simulink model "LTI_Unmodeled_test"  (Simulink 7.3)
settings: Solver=ode45  StartTime=0.0  StopTime=10.0  RelTol=1e-3
settings Model: Creator=MD710  LastModifiedBy=MD710
settings DebuggingCC: SaveWithParameterizedLinksMsg=none  SolverPrmCheckMsg=none  MultiTaskDSMMsg=warning  MultiTaskCondExecSysMsg=none  FcnCallInpInsideContextMsg=Enable All  StrictBusMsg=None
settings HardwareCC: TargetHWDeviceType=32-bit Generic
settings RTWCC: IncludeERTFirstTime=on
settings GRTTargetCC: TargetFcnLib=ansi_tfl_tmw.mat

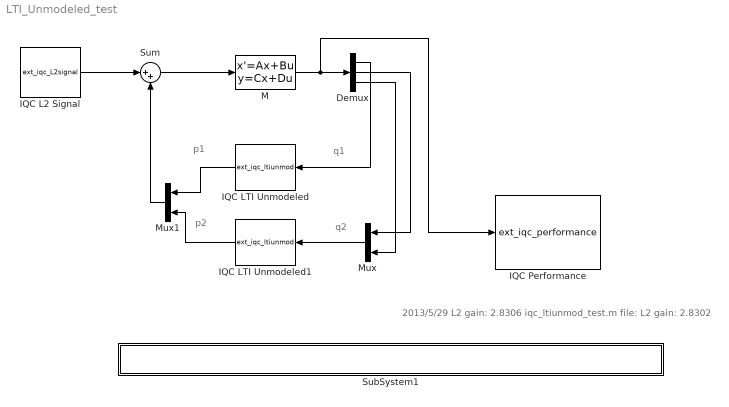
== system LTI_Unmodeled_test ==
  note: p1
  note: q1
  note: q2
  note: p2
  note: 2013/5/29 L2 gain: 2.8306
      | iqc_ltiunmod_test.m file: L2 gain: 2.8302
  Demux : Demux  Outputs=3
  IQC L2 Signal : M-S-Function  FunctionName=ext_iqc_L2signal  Parameters=sig_size,sam_time,sig_type,tru_time,sig_amp,sig_fre,user_cus  mask(IQC L2 signal(ver:0.1)){sig_size=2, sam_time=0, sig_type=Step, tru_time=10, sig_amp=1, sig_fre=1, user_cus='2*exp(3*t)'}
      mask prompts: sig_size "Signal Dimension:(Default: 1)"; sam_time "Sample Time:(Default: 0)"; sig_type "Signal Type:"; tru_time "Truncation Time:"; sig_amp "Maximum Amplitude:"; sig_fre "Frequency:"; user_cus "Custom:"
      mask help:
      | Important:
      | In IQC procedure step (as commond iqc_gain_tbx, the task is get
      | L2 gain value), regardless of the user to choose which option (ex sine...),
      | here regarded as generalized L2 signal.
      mask StyleString: edit,edit,popup(Step|Square wave|Sine wave|Custom|Random|External),edit,edit,edit,edit
      mask CallbackString: ||iqc_block_cho(gcb,'L2signal_type')||||
      mask TabNameString: Generalized Parameters,Generalized Parameters,Simulink Parameters,Simulink Parameters,Simulink Parameters,Simulink Parameters,Simulink Parameters
      mask Display: plot(0:0.1:10,[sin(0:0.1:6.2) zeros(1,38)])
  IQC LTI Unmodeled : M-S-Function  FunctionName=ext_iqc_ltiunmod  Parameters=pole,out_dim,upp_bou,out_var  mask(IQC LTI Unmodeled(ver:0.1)){pole=4, out_dim=1, upp_bou=1, out_var=''}
      mask prompts: pole "Pole:(Default: [1])"; out_dim "The Dimension of The Output Signal:(Default: -1)"; upp_bou "Upper Bound of The H-inf norm of delta:(Default: 1)"; out_var "Output Variable:(Default: empty)"
      mask help:
      | Example: [w,X]=iqc_ltiunmod(v,a,n,g)
      | Pole:
      |      [a]
      | The Dimension of The Output Signal:
      |       n
      | Upper Bound of The H-inf norm of delta:
      |       g
      | Output Variable:
      |      {'X'}
      mask Help: eval('doc iqc_ltiunmod')
      mask Display: disp('\fontsize{16}\Delta(S)', 'texmode','on');
  IQC LTI Unmodeled1 : M-S-Function  FunctionName=ext_iqc_ltiunmod  Parameters=pole,out_dim,upp_bou,out_var  mask(IQC LTI Unmodeled(ver:0.1)){pole=4, out_dim=1, upp_bou=1, out_var=''}
      mask prompts: pole "Pole:(Default: [1])"; out_dim "The Dimension of The Output Signal:(Default: -1)"; upp_bou "Upper Bound of The H-inf norm of delta:(Default: 1)"; out_var "Output Variable:(Default: empty)"
      mask help:
      | Example: [w,X]=iqc_ltiunmod(v,a,n,g)
      | Pole:
      |      [a]
      | The Dimension of The Output Signal:
      |       n
      | Upper Bound of The H-inf norm of delta:
      |       g
      | Output Variable:
      |      {'X'}
      mask Help: eval('doc iqc_ltiunmod')
      mask Display: disp('\fontsize{16}\Delta(S)', 'texmode','on');
  IQC Performance : M-S-Function  FunctionName=ext_iqc_performance  Parameters=imp_met,save_lin_com,isiqcbode,fre_ran,uselmitool,lmi_par  mask(IQC Performance(ver:0.1)){imp_met=Only Calculation, save_lin_com=off, isiqcbode=off, fre_ran='', uselmitool=lmilab, lmi_par=''}
      mask prompts: imp_met "Implementation Methods"; save_lin_com "Save the Linear File and Command File"; isiqcbode "Display IQC Bode Figure"; fre_ran "Frequency Range:(Default: empty)"; uselmitool "LMI Tool:"; lmi_par "Parameter:(if empty use define)"
      mask help:
      | Important:
      | In IQC toolbox calculate step (as commond iqc_gain_tbx, the task is get
      | L2 gain value), regardless of the user to connect any signal input(Even if
      | not a signal), here regarded as generalized L2 signal.
      |
      | Example 1: setlmioptions('',[0 200 0 0 777])
      | the block parameter is
      | LMI Tool: lmilab
      | Parameter:
      |        [0 200 0 0 777]
      |
      | Example 2: setlmioptions('yalmip','solver','sdpt3','verbose',1)
      | the block parameter is
      | LMI Tool: yalmip
      | Parameter:
      |        {'solver',sdpt3','verbose',1}
      mask Help:
      | <a href="matlab:doc abst_init_iqc;">abst_init_iqc</a>
      | <a href="matlab:doc setlmioptions;">setlmioptions</a>
      | <a href="matlab:doc iqc_gain_tbx;">iqc_gain_tbx</a>
      mask StyleString: popup(Calculation and Simulation|Only Calculation|Only Simulation),checkbox,checkbox,edit,popup(lmilab|yalmip),edit
      mask CallbackString: iqc_block_cho(gcb,'performance_imp')||iqc_block_cho(gcb,'performance_bodefre')|||
      mask TabNameString: Parameter,Parameter,Parameter,Parameter,LMI Parameter,LMI Parameter
      mask Display: fprintf('In -> Out \n performance \n L2 gain:\n%4.4f',2.8306);
  M : StateSpace  A=[-100 0 0 0;0 -80 0 0;0 0 -10 0;0 0 0 -8]  B=[8 0;8 0;2 0;0 2]  C=[-8.333 0 0 0;0 -6.667 0 0;0 0 3.333 2.667]  D=[0.6667 0;0.6667 0;0 0]
  Mux : Mux  Inputs=2
  Mux1 : Mux  Inputs=2
  SubSystem1 : Subsystem  mask{filename=iqc_ltiunmod_test.m}
      mask init:
      | x_dir=which(filename);
      | x=x_dir;
      settings: OpenFcn=|
      | x_dir=which('iqc_ltiunmod_test.m');
      | x=x_dir;
      | edit(x);
      mask Display: disp(['MATLAB file: ' x]);
  Sum : Sum  Inputs=|++
  wires:
  IQC L2 Signal/1 -> Sum/1
  Sum/1 -> M/1
  M/1 -> IQC Performance/1, Demux/1
  Demux/1 -> IQC LTI Unmodeled/1
  Demux/2 -> Mux/1
  Demux/3 -> Mux/2
  Mux/1 -> IQC LTI Unmodeled1/1
  IQC LTI Unmodeled/1 -> Mux1/1
  IQC LTI Unmodeled1/1 -> Mux1/2
  Mux1/1 -> Sum/2

== system LTI_Unmodeled_test/SubSystem1 ==
